simulink model "cap_eq_circuit_pascal5_single_shot"  (R2019a)
settings: Solver=FixedStepAuto  StartTime=0.0  StopTime=sim_time  FixedStep=resolution  MinStep=0.001  RelTol=1e-4  EnableMultiTasking=on
values from neighbouring files (symbols this model uses):
  amps_in = double(amps_in)    [ClassHybrid.m]    (also in Sc.m = double(amps_in_); workspace_test_model.mat = 0)
  capacitance = double(obj.farads)    [ClassHybrid.m]    (also in Sc.m; workspace_test_model.mat = 5)
  resolution = double(resolution)    [ClassHybrid.m]    (also in Sc.m = double(resolution_); matlab.mat = 1; model_out_all.mat = 0.5; workspace_test_model.mat = 10)
  tStep = resolution    (= 0.1)    [ClassHybrid.m]    (also in Sc.m; matlab.mat = 10; model_out_all.mat = 1; raw.mat = 1)
  v_init = ones(x(1), 1, nSeries)    [ClassHybrid.m]    (also in Sc.m; workspace_test_model.mat = [4 4 4 4 4 4 4 4 4 4 4 4 ... (15 elements, 1x5x3)])
libraries: powerlib x127, simulink x5
(part 1 of 2)
settings Model: Creator=ttsh  LastModifiedBy=ttsh
settings SolverCC: ZeroCrossAlgorithm=Adaptive  SolverResetMethod=Robust
settings DataIOCC: LimitDataPoints=on  SaveFormat=Array  ReturnWorkspaceOutputs=off
settings OptimizationCC: LifeSpan=inf
settings DebuggingCC: SolverPrmCheckMsg=warning  UniqueDataStoreMsg=error  AllowSymbolicDim=off  SFUnexpectedBacktrackingDiag=warning  SFNoUnconditionalDefaultTransitionDiag=warning  SFExecutionAtInitializationDiag=none  ArithmeticOperatorsInVariantConditions=warning
settings HardwareCC: ProdBitPerPointer=32  ProdBitPerSizeT=32  ProdBitPerPtrDiffT=32  ProdLargestAtomicFloat=None  ProdIntDivRoundTo=Undefined  ProdEndianess=Unspecified  ProdWordSize=32  ProdHWDeviceType=32-bit Generic
settings ModelReferenceCC: PropagateSignalLabelsOutOfModel=off
settings SFSimCC: SimUseLocalCustomCode=off
settings RTWCC: RTWUseLocalCustomCode=off
settings CodeAppCC: StateflowObjectComments=on
settings GRTTargetCC: TargetLangStandard=C89/C90 (ANSI)  GeneratePreprocessorConditionals=Disable all
settings ConfigComp: CovMetricSettings=dw  CovHtmlReporting=on  CovSaveCumulativeToWorkspaceVar=on  CovSaveSingleToWorkspaceVar=on  CovExternalEMLEnable=off  CovSFcnEnable=off
settings SimscapeCC: SimscapeNormalizeSystem=off

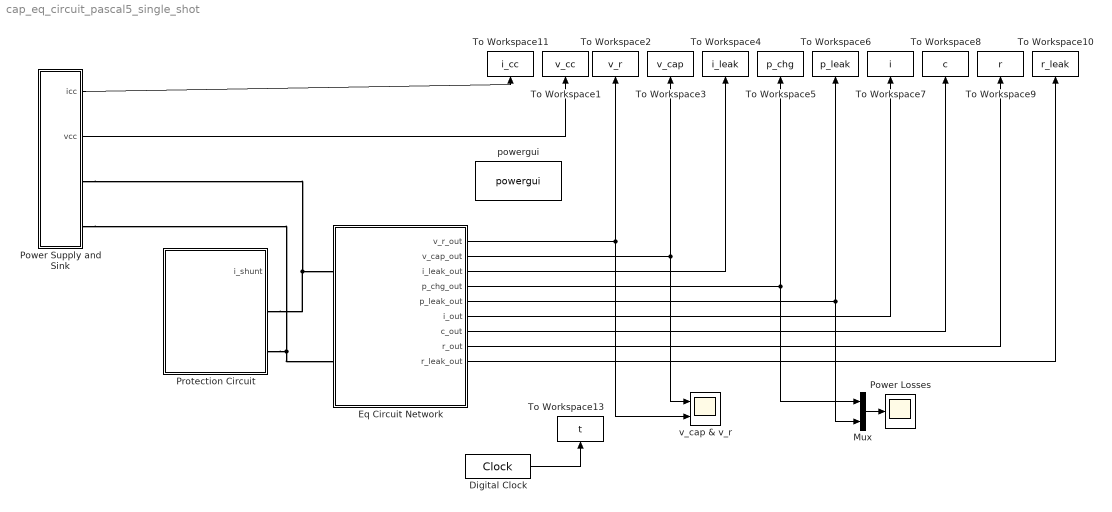
== system cap_eq_circuit_pascal5_single_shot ==
  Digital Clock : DigitalClock  SampleTime=resolution
  Eq Circuit Network : Subsystem  mask{r_leak=inf, c=capacitance, r_esr=0.01, ord=5, v_init1=v_init(1), v_init2=v_init(2), v_init3=v_init(3), v_init4=v_init(4), v_init5=v_init(5)}
      mask prompts: r_leak "R Leak /ohm (inf for disabled)"; c "Capacitance /F"; r_esr "ESR"; ord "Elements (pascal order)"; v_init1 "Initial capacitor voltage"; v_init2 "Initial capacitor voltage"; v_init3 "Initial capacitor voltage"; v_init4 "Initial capacitor voltage"; v_init5 "Initial capacitor voltage"
  Mux : Mux  Inputs=2
  Power Losses : Scope
  Power Supply and Sink : Subsystem  mask{v_ovp=24}
      mask prompts: v_ovp "V OVP"
  Protection Circuit : Subsystem  mask{r=1, d=0.01, v_cut=8.1, v_min=0}
      mask prompts: r "Series resistance"; d "Rate limit"; v_cut "v cutoff"; v_min "v min"
  To Workspace1 : ToWorkspace  VariableName=v_cc  SampleTime=-1
      settings: Save2DSignal=2-D array (concatenate along first dimension)
  To Workspace10 : ToWorkspace  VariableName=r_leak  SampleTime=-1
  To Workspace11 : ToWorkspace  VariableName=i_cc  SampleTime=-1
      settings: Save2DSignal=2-D array (concatenate along first dimension)
  To Workspace13 : ToWorkspace  VariableName=t  SampleTime=-1
      settings: Save2DSignal=2-D array (concatenate along first dimension)
  To Workspace2 : ToWorkspace  VariableName=v_r  SampleTime=-1
  To Workspace3 : ToWorkspace  VariableName=v_cap  SampleTime=-1
  To Workspace4 : ToWorkspace  VariableName=i_leak  SampleTime=-1
  To Workspace5 : ToWorkspace  VariableName=p_chg  SampleTime=-1
  To Workspace6 : ToWorkspace  VariableName=p_leak  SampleTime=-1
  To Workspace7 : ToWorkspace  VariableName=i  SampleTime=-1
  To Workspace8 : ToWorkspace  VariableName=c  SampleTime=-1
  To Workspace9 : ToWorkspace  VariableName=r  SampleTime=-1
  powergui : powerlib/powergui  Priority=1  SimulationMode=Discrete  SampleTime=tStep  frequency=60  Iterations=50  frequencyindice=0  Pbase=100e6  ErrMax=1e-4  UnitsV=V  UnitsW=W  buscounter=0  FunctionMessages=off  echomessages=off  EnableUseOfTLC=off  CurrentSourceSwitches=on  DisableSnubberDevices=on  DisableRonSwitches=off  DisableVfSwitches=off  DisplayEquations=off  AutomaticDiscreteSolvers=off  SolverType=Tustin  Interpol=off  ExternalGateDelay=off  methode=off  Ts=0  x0status=blocks  SPID=on  SwTol=0  HookPort=off  NonlinearTolerance=0  nMaxIteration=15  ContinueOnMaxIteration=off  RestoreLinks=warning  ResistiveCurrentMeasurement=off  Frange=[0:2:500]  Ylog=off  Xlog=on  ShowGrid=off  save=off  variable=ZData  structure=0  ZoomFFT=off  StartTime=0.0  cycles=1  DisplayStyle=1  fundamental=60  FreqAxis=off  MaxFrequency=1000  frequencyindicesteady=1  RmsSteady=1  display=off
      settings: SourceProductName=Simscape Electrical
  v_cap & v_r : Scope  NumInputPorts=2
  wires:
  Eq Circuit Network/1(v_r_out) -> v_cap & v_r/2, To Workspace2/1
  Eq Circuit Network/2(v_cap_out) -> v_cap & v_r/1, To Workspace3/1
  Eq Circuit Network/3(i_leak_out) -> To Workspace4/1
  Eq Circuit Network/4(p_chg_out) -> Mux/1, To Workspace5/1
  Eq Circuit Network/5(p_leak_out) -> Mux/2, To Workspace6/1
  Eq Circuit Network/6(i_out) -> To Workspace7/1
  Eq Circuit Network/7(c_out) -> To Workspace8/1
  Eq Circuit Network/8(r_out) -> To Workspace9/1
  Eq Circuit Network/9(r_leak_out) -> To Workspace10/1
  Mux/1 -> Power Losses/1
  Power Supply and Sink/1(icc) -> To Workspace11/1
  Power Supply and Sink/2(vcc) -> To Workspace1/1
  Digital Clock/1 -> To Workspace13/1
  connections:
  Power Supply and Sink/RConn1 -- Protection Circuit/RConn1 -- Eq Circuit Network/LConn1
  Power Supply and Sink/RConn2 -- Protection Circuit/RConn2 -- Eq Circuit Network/LConn2

== system cap_eq_circuit_pascal5_single_shot/Eq Circuit Network ==
  note: 6x 700R
  note: 4x 1k4
  note: 4x 625R
  note: 1x 550R
  note: 1x 4k
  Subsystem : Subsystem  mask{c=c, r_esr=625, r_leak=r_leak, v_init=v_init2}
      mask prompts: c "Capacitance /F"; r_esr "Series resistance /ohm"; r_leak "Leak resistance /ohm (inf for disabled)"; v_init "Initial capacitor voltage"
  Subsystem1 : Subsystem  mask{c=c, r_esr=1.4e3, r_leak=r_leak, v_init=v_init4}
      mask prompts: c "Capacitance /F"; r_esr "Series resistance /ohm"; r_leak "Leak resistance /ohm (inf for disabled)"; v_init "Initial capacitor voltage"
  Subsystem2 : Subsystem  mask{c=c, r_esr=700, r_leak=r_leak, v_init=v_init3}
      mask prompts: c "Capacitance /F"; r_esr "Series resistance /ohm"; r_leak "Leak resistance /ohm (inf for disabled)"; v_init "Initial capacitor voltage"
  Subsystem5 : Subsystem  mask{c=c, r_esr=4e3, r_leak=r_leak, v_init=v_init5}
      mask prompts: c "Capacitance /F"; r_esr "Series resistance /ohm"; r_leak "Leakage resistance /ohm (inf for disabled)"; v_init "Initial capacitor voltage"
  Subsystem8 : Subsystem  mask{c=c, r_esr=550, r_leak=r_leak, v_init=v_init1}
      mask prompts: c "Capacitance /F"; r_esr "Series resistance /ohm"; r_leak "Leakage resistance /ohm (inf for disabled)"; v_init "Initial capacitor voltage"
  VCC_in : PMIOPort  Side=Left
  VSS_in : PMIOPort  Port=2  Side=Left
  VCC_out : PMIOPort  Port=3  Side=Right
  VSS_out : PMIOPort  Port=4  Side=Right
  v_r_out : Outport
  v_cap_out : Outport  Port=2
  i_leak_out : Outport  Port=3
  p_chg_out : Outport  Port=4
  p_leak_out : Outport  Port=5
  i_out : Outport  Port=6
  c_out : Outport  Port=7
  r_out : Outport  Port=8
  r_leak_out : Outport  Port=9
  wires:
  Subsystem5/5(p_leak_out) -> p_leak_out/1
  Subsystem5/6(i_out) -> i_out/1
  Subsystem5/4(p_chg_out) -> p_chg_out/1
  Subsystem5/7(c_out) -> c_out/1
  Subsystem5/3(i_leak_out) -> i_leak_out/1
  Subsystem5/8(r_out) -> r_out/1
  Subsystem5/2(v_cap_out) -> v_cap_out/1
  Subsystem5/9(r_leak_out) -> r_leak_out/1
  Subsystem5/1(v_r_out) -> v_r_out/1
  Subsystem8/3(i_leak_out) -> Subsystem/3(In3)
  Subsystem8/6(i_out) -> Subsystem/6(In6)
  Subsystem8/9(r_leak_out) -> Subsystem/9(In9)
  Subsystem8/4(p_chg_out) -> Subsystem/4(In4)
  Subsystem8/10(l_out) -> Subsystem/10(In10)
  Subsystem8/8(r_out) -> Subsystem/8(In8)
  Subsystem8/5(p_leak_out) -> Subsystem/5(In5)
  Subsystem8/7(c_out) -> Subsystem/7(In7)
  Subsystem8/1(v_r_out) -> Subsystem/1(In1)
  Subsystem8/2(v_cap_out) -> Subsystem/2(In2)
  Subsystem1/6(Out6) -> Subsystem5/6(i_in)
  Subsystem1/8(Out8) -> Subsystem5/8(r_in)
  Subsystem1/4(Out4) -> Subsystem5/4(p_chg_in)
  Subsystem1/7(Out7) -> Subsystem5/7(c_in)
  Subsystem1/9(Out9) -> Subsystem5/9(r_leak_in)
  Subsystem1/3(Out3) -> Subsystem5/3(i_leak_in)
  Subsystem1/10(Out10) -> Subsystem5/10(l_in)
  Subsystem1/5(Out5) -> Subsystem5/5(p_leak_in)
  Subsystem1/2(Out2) -> Subsystem5/2(v_cap_in)
  Subsystem1/1(Out1) -> Subsystem5/1(v_r_in)
  Subsystem/3(Out3) -> Subsystem2/3(In3)
  Subsystem/10(Out10) -> Subsystem2/10(In10)
  Subsystem/8(Out8) -> Subsystem2/8(In8)
  Subsystem/1(Out1) -> Subsystem2/1(In1)
  Subsystem/2(Out2) -> Subsystem2/2(In2)
  Subsystem/6(Out6) -> Subsystem2/6(In6)
  Subsystem/9(Out9) -> Subsystem2/9(In9)
  Subsystem/7(Out7) -> Subsystem2/7(In7)
  Subsystem/4(Out4) -> Subsystem2/4(In4)
  Subsystem/5(Out5) -> Subsystem2/5(In5)
  Subsystem2/5(Out5) -> Subsystem1/5(In5)
  Subsystem2/8(Out8) -> Subsystem1/8(In8)
  Subsystem2/6(Out6) -> Subsystem1/6(In6)
  Subsystem2/2(Out2) -> Subsystem1/2(In2)
  Subsystem2/10(Out10) -> Subsystem1/10(In10)
  Subsystem2/9(Out9) -> Subsystem1/9(In9)
  Subsystem2/1(Out1) -> Subsystem1/1(In1)
  Subsystem2/3(Out3) -> Subsystem1/3(In3)
  Subsystem2/4(Out4) -> Subsystem1/4(In4)
  Subsystem2/7(Out7) -> Subsystem1/7(In7)
  connections:
  Subsystem8/LConn1 -- VCC_in/RConn1
  VSS_in/RConn1 -- Subsystem8/LConn2
  Subsystem8/RConn2 -- Subsystem/LConn2
  Subsystem8/RConn1 -- Subsystem/LConn1
  Subsystem1/RConn2 -- Subsystem5/LConn2
  Subsystem1/RConn1 -- Subsystem5/LConn1
  Subsystem/RConn1 -- Subsystem2/LConn1
  Subsystem/RConn2 -- Subsystem2/LConn2
  Subsystem1/LConn2 -- Subsystem2/RConn2
  Subsystem1/LConn1 -- Subsystem2/RConn1
  VCC_out/RConn1 -- Subsystem5/RConn1
  Subsystem5/RConn2 -- VSS_out/RConn1

== system cap_eq_circuit_pascal5_single_shot/Power Supply and Sink ==
  Compare To Zero : simulink/Logic and Bit Operations/Compare To Zero  relop=>  OutDataTypeStr=boolean
  Compare To Zero1 : simulink/Logic and Bit Operations/Compare To Zero  relop=~=  OutDataTypeStr=boolean
  Constant : Constant  Value=3*5
  Constant1 : Constant  Value=amps_in
  Controlled Current Source2 : powerlib/Electrical Sources/Controlled Current Source  Initialize=on  Source_Type=DC  Amplitude=0  Phase=0  Frequency=0  Measurements=None
      settings: SourceProductName=Simscape Electrical
  Discrete PID Controller : simulink/Continuous/PID Controller  Controller=PI  Form=Parallel  TimeDomain=Discrete-time  SampleTime=-1  IntegratorMethod=Forward Euler  FilterMethod=Forward Euler  ControllerParametersSource=internal  P=1  I=0.02  D=0  UseFilter=on  N=100  TunerSelectOption=Transfer Function Based (PID Tuner App)  InitialConditionSource=internal  InitialConditionForIntegrator=0  InitialConditionForFilter=0  DifferentiatorICPrevScaledInput=0  ExternalReset=none  TrackingMode=off  Kt=1  LimitOutput=on  UpperSaturationLimit=0.1  LowerSaturationLimit=0  LinearizeAsGain=off  AntiWindupMode=none  Kb=1  POutMin=[]  POutMax=[]  IOutMin=[]  IOutMax=[]  DOutMin=[]  DOutMax=[]  NOutMin=[]  NOutMax=[]  SumOutMin=[]  SumOutMax=[]  SaturationOutMin=[]  SaturationOutMax=[]  PParamMin=[]  PParamMax=[]  IParamMin=[]  IParamMax=[]  DParamMin=[]  DParamMax=[]  NParamMin=[]  NParamMax=[]  KbParamMin=[]  KbParamMax=[]  KtParamMin=[]  KtParamMax=[]  KbOutMin=[]  KbOutMax=[]  KtOutMin=[]  KtOutMax=[]  IntegratorOutMin=[]  IntegratorOutMax=[]  FilterOutMin=[]  FilterOutMax=[]  SumI1OutMin=[]  SumI1OutMax=[]  SumI2OutMin=[]  SumI2OutMax=[]  SumI3OutMin=[]  SumI3OutMax=[]  SumI4OutMin=[]  SumI4OutMax=[]  SumDOutMin=[]  SumDOutMax=[]  DifferentiatorOutMin=[]  DifferentiatorOutMax=[]  FilterDiffOutCoefMin=[]  FilterDiffOutCoefMax=[]  ReciprocalOutMin=[]  ReciprocalOutMax=[]  SumDenOutMin=[]  SumDenOutMax=[]  SumNumOutMin=[]  SumNumOutMax=[]  DivideOutMin=[]  DivideOutMax=[]  IntegratorContinuousStateAttributes=''  IntegratorStateMustResolveToSignalObject=off  IntegratorRTWStateStorageClass=Auto  FilterContinuousStateAttributes=''  FilterStateMustResolveToSignalObject=off  FilterRTWStateStorageClass=Auto  ParallelPVariant=InternalParameters  IdealPVariant=Disabled  IVariant=InternalParameters  DVariant=Disabled  IntegratorVariant=Discrete  SatVariant=Enabled  AWVariant=Passthrough  PCopyVariant=Disabled  TRVariant=Disabled  FdbkBlocksVariant=Forward  IdealPFdbkVariant=Disabled  SatFdbkVariant=Disabled  DerivativeFilterVariant=Disabled  NVariant=Disabled  NCopyVariant=Disabled_SignalSpec  FilterICVariant=Disabled  IntegratorICVariant=InternalICs  ExternalResetVariant=Disabled  TRSumVariant=Passthrough  SumFdbkVariant=Disabled  SumVariant=Sum_PI
  Display : Display
  Memory : Memory  InitialCondition=1  InheritSampleTime=on  LinearizeAsDelay=on
  Mosfet : powerlib/Power Electronics/Mosfet  Ron=0.1  Lon=0  Rd=0.01  Vfd=0  IC=0  Rs=1e5  Cs=inf  Measurements=off
      settings: SourceProductName=Simscape Electrical
  Mosfet1 : powerlib/Power Electronics/Mosfet  Ron=0.1  Lon=0  Rd=0.01  Vfd=0  IC=0  Rs=1e5  Cs=inf  Measurements=off
      settings: SourceProductName=Simscape Electrical
  Saturation : Saturate  UpperLimit=inf  LowerLimit=0
  Series RLC Branch : powerlib/Elements/Series RLC Branch  LConnTagsString=__new0  RConnTagsString=__new0  BranchType=R  Resistance=0.001  Inductance=1e-9  SetiL0=off  InitialCurrent=0  Capacitance=1e-6  Setx0=off  InitialVoltage=0  Measurements=None
      settings: SourceProductName=Simscape Electrical
  Series RLC Branch1 : powerlib/Elements/Series RLC Branch  LConnTagsString=__new0  RConnTagsString=__new0  BranchType=R  Resistance=1e9  Inductance=1e-9  SetiL0=off  InitialCurrent=0  Capacitance=1e-6  Setx0=off  InitialVoltage=0  Measurements=None
      settings: SourceProductName=Simscape Electrical
  Series RLC Branch2 : powerlib/Elements/Series RLC Branch  LConnTagsString=__new0  RConnTagsString=__new0  BranchType=R  Resistance=1e9  Inductance=1e-9  SetiL0=off  InitialCurrent=0  Capacitance=1e-6  Setx0=off  InitialVoltage=0  Measurements=None
      settings: SourceProductName=Simscape Electrical
  Sum : Sum  Inputs=|-+
  Switch : Switch  Criteria=u2 > Threshold
  i_cc : powerlib/Measurements/Current Measurement  PhasorSimulation=off  OutputType=Complex  PSBequivalent=0
      settings: SourceProductName=Simscape Electrical
  v_cap_single1 : powerlib/Measurements/Voltage Measurement  PhasorSimulation=off  OutputType=Complex  PSBequivalent=0
      settings: SourceProductName=Simscape Electrical
  V_cc : PMIOPort  Side=Right
  V_ss : PMIOPort  Port=2  Side=Right
  icc : Outport
  vcc : Outport  Port=2
  wires:
  Saturation/1 -> Switch/3
  Compare To Zero1/1 -> Mosfet1/1, Mosfet/1
  i_cc/1 -> icc/1
  v_cap_single1/1 -> vcc/1, [vcc]
  [vcc] -> Sum/1, Compare To Zero/1
  Memory/1 -> Switch/2
  Compare To Zero/1 -> Memory/1
  Switch/1 -> Controlled Current Source2/1
  Sum/1 -> Discrete PID Controller/1
  Constant1/1 -> Saturation/1, Compare To Zero1/1, Switch/1
  Constant/1 -> Sum/2
  Discrete PID Controller/1 -> Display/1
  connections:
  Mosfet/LConn1 -- Mosfet1/LConn1
  Mosfet1/RConn1 -- Series RLC Branch2/LConn1 -- Controlled Current Source2/RConn1
  i_cc/LConn1 -- V_cc/RConn1
  i_cc/RConn1 -- Mosfet/RConn1 -- Series RLC Branch1/LConn1 -- v_cap_single1/LConn1
  Controlled Current Source2/LConn1 -- Series RLC Branch/LConn1
  v_cap_single1/LConn2 -- Series RLC Branch2/RConn1 -- Series RLC Branch/RConn1 -- Series RLC Branch1/RConn1 -- V_ss/RConn1

== system cap_eq_circuit_pascal5_single_shot/Protection Circuit ==
  note: 10nF
  Compare To Constant : simulink/Logic and Bit Operations/Compare To Constant  relop=>  const=v_cut  OutDataTypeStr=boolean
  Compare To Constant1 : simulink/Logic and Bit Operations/Compare To Constant  relop=<  const=v_min  OutDataTypeStr=boolean
  Mosfet : powerlib/Power Electronics/Mosfet  Ron=0.1  Lon=0  Rd=0.01  Vfd=0  IC=0  Rs=1e5  Cs=inf  Measurements=off
      settings: SourceProductName=Simscape Electrical
  Mosfet1 : powerlib/Power Electronics/Mosfet  Ron=0.1  Lon=0  Rd=0.01  Vfd=0  IC=0  Rs=1e5  Cs=inf  Measurements=off
      settings: SourceProductName=Simscape Electrical
  Parallel RLC Branch11 : powerlib/Elements/Parallel RLC Branch  LConnTagsString=a  RConnTagsString=__new0  BranchType=C  Resistance=1  Inductance=1e-3  SetiL0=off  InitialCurrent=0  Capacitance=0.00000001  Setx0=on  InitialVoltage=1.0  Measurements=None
      settings: SourceProductName=Simscape Electrical
  Series RLC Branch1 : powerlib/Elements/Series RLC Branch  LConnTagsString=__new0  RConnTagsString=__new0  BranchType=R  Resistance=r  Inductance=1e-3  SetiL0=off  InitialCurrent=0  Capacitance=1e-6  Setx0=off  InitialVoltage=0  Measurements=None
      settings: SourceProductName=Simscape Electrical
  Sum : Sum  Inputs=++|
  i_cc : powerlib/Measurements/Current Measurement  PhasorSimulation=off  OutputType=Complex  PSBequivalent=0
      settings: SourceProductName=Simscape Electrical
  v_cap_single2 : powerlib/Measurements/Voltage Measurement  PhasorSimulation=off  OutputType=Complex  PSBequivalent=0
      settings: SourceProductName=Simscape Electrical
  vcc : PMIOPort  Side=Right
  vss : PMIOPort  Port=2  Side=Right
  i_shunt : Outport
  wires:
  i_cc/1 -> i_shunt/1
  v_cap_single2/1 -> Compare To Constant1/1, Compare To Constant/1
  Compare To Constant/1 -> Sum/2
  Compare To Constant1/1 -> Sum/1
  Sum/1 -> Mosfet/1, Mosfet1/1
  connections:
  Series RLC Branch1/LConn1 -- i_cc/LConn1
  i_cc/RConn1 -- Mosfet/RConn1
  Mosfet1/LConn1 -- Mosfet/LConn1
  vcc/RConn1 -- Mosfet1/RConn1 -- Parallel RLC Branch11/LConn1 -- v_cap_single2/LConn1
  v_cap_single2/LConn2 -- Parallel RLC Branch11/RConn1 -- vss/RConn1 -- Series RLC Branch1/RConn1

== system cap_eq_circuit_pascal5_single_shot/Eq Circuit Network/Subsystem ==
  In1 : Inport
  In2 : Inport  Port=2
  In3 : Inport  Port=3
  In4 : Inport  Port=4
  In5 : Inport  Port=5
  In6 : Inport  Port=6
  In7 : Inport  Port=7
  In8 : Inport  Port=8
  In9 : Inport  Port=9
  In10 : Inport  Port=10
  Subsystem1 : Subsystem  mask{c=c, r_esr=r_esr, r_leak=r_leak, v_init=v_init}
      mask prompts: c "Capacitance /F"; r_esr "Series resistance /ohm"; r_leak "Leakage resistance /ohm (inf for disabled)"; v_init "Initial capacitor voltage"
  Subsystem2 : Subsystem  mask{c=c, r_esr=r_esr, r_leak=r_leak, v_init=v_init}
      mask prompts: c "Capacitance /F"; r_esr "Series resistance /ohm"; r_leak "Leakage resistance /ohm (inf for disabled)"; v_init "Initial capacitor voltage"
  Subsystem3 : Subsystem  mask{c=c, r_esr=r_esr, r_leak=r_leak, v_init=v_init}
      mask prompts: c "Capacitance /F"; r_esr "Series resistance /ohm"; r_leak "Leakage resistance /ohm (inf for disabled)"; v_init "Initial capacitor voltage"
  Subsystem5 : Subsystem  mask{c=c, r_esr=r_esr, r_leak=r_leak, v_init=v_init}
      mask prompts: c "Capacitance /F"; r_esr "Series resistance /ohm"; r_leak "Leakage resistance /ohm (inf for disabled)"; v_init "Initial capacitor voltage"
  Conn1 : PMIOPort  Side=Left
  Conn2 : PMIOPort  Port=2  Side=Right
  Conn3 : PMIOPort  Port=3  Side=Left
  Conn4 : PMIOPort  Port=4  Side=Right
  Out1 : Outport
  Out2 : Outport  Port=2
  Out3 : Outport  Port=3
  Out4 : Outport  Port=4
  Out5 : Outport  Port=5
  Out6 : Outport  Port=6
  Out7 : Outport  Port=7
  Out8 : Outport  Port=8
  Out9 : Outport  Port=9
  Out10 : Outport  Port=10
  wires:
  In8/1 -> Subsystem5/8(r_in)
  In3/1 -> Subsystem5/3(i_leak_in)
  In10/1 -> Subsystem5/10(l_in)
  In1/1 -> Subsystem5/1(v_r_in)
  In7/1 -> Subsystem5/7(c_in)
  In4/1 -> Subsystem5/4(p_chg_in)
  In5/1 -> Subsystem5/5(p_leak_in)
  In6/1 -> Subsystem5/6(i_in)
  In9/1 -> Subsystem5/9(r_leak_in)
  In2/1 -> Subsystem5/2(v_cap_in)
  Subsystem5/1(v_r_out) -> Subsystem1/1(v_r_in)
  Subsystem5/2(v_cap_out) -> Subsystem1/2(v_cap_in)
  Subsystem5/3(i_leak_out) -> Subsystem1/3(i_leak_in)
  Subsystem5/4(p_chg_out) -> Subsystem1/4(p_chg_in)
  Subsystem5/5(p_leak_out) -> Subsystem1/5(p_leak_in)
  Subsystem5/6(i_out) -> Subsystem1/6(i_in)
  Subsystem5/7(c_out) -> Subsystem1/7(c_in)
  Subsystem5/8(r_out) -> Subsystem1/8(r_in)
  Subsystem5/9(r_leak_out) -> Subsystem1/9(r_leak_in)
  Subsystem5/10(l_out) -> Subsystem1/10(l_in)
  Subsystem1/1(v_r_out) -> Subsystem2/1(v_r_in)
  Subsystem1/2(v_cap_out) -> Subsystem2/2(v_cap_in)
  Subsystem1/3(i_leak_out) -> Subsystem2/3(i_leak_in)
  Subsystem1/4(p_chg_out) -> Subsystem2/4(p_chg_in)
  Subsystem1/5(p_leak_out) -> Subsystem2/5(p_leak_in)
  Subsystem1/6(i_out) -> Subsystem2/6(i_in)
  Subsystem1/7(c_out) -> Subsystem2/7(c_in)
  Subsystem1/8(r_out) -> Subsystem2/8(r_in)
  Subsystem1/9(r_leak_out) -> Subsystem2/9(r_leak_in)
  Subsystem1/10(l_out) -> Subsystem2/10(l_in)
  Subsystem2/1(v_r_out) -> Subsystem3/1(v_r_in)
  Subsystem3/1(v_r_out) -> Out1/1
  Subsystem2/2(v_cap_out) -> Subsystem3/2(v_cap_in)
  Subsystem2/3(i_leak_out) -> Subsystem3/3(i_leak_in)
  Subsystem2/4(p_chg_out) -> Subsystem3/4(p_chg_in)
  Subsystem2/5(p_leak_out) -> Subsystem3/5(p_leak_in)
  Subsystem2/6(i_out) -> Subsystem3/6(i_in)
  Subsystem2/7(c_out) -> Subsystem3/7(c_in)
  Subsystem2/8(r_out) -> Subsystem3/8(r_in)
  Subsystem2/9(r_leak_out) -> Subsystem3/9(r_leak_in)
  Subsystem2/10(l_out) -> Subsystem3/10(l_in)
  Subsystem3/2(v_cap_out) -> Out2/1
  Subsystem3/3(i_leak_out) -> Out3/1
  Subsystem3/4(p_chg_out) -> Out4/1
  Subsystem3/5(p_leak_out) -> Out5/1
  Subsystem3/6(i_out) -> Out6/1
  Subsystem3/7(c_out) -> Out7/1
  Subsystem3/8(r_out) -> Out8/1
  Subsystem3/9(r_leak_out) -> Out9/1
  Subsystem3/10(l_out) -> Out10/1
  connections:
  Subsystem5/LConn2 -- Conn3/RConn1
  Subsystem5/LConn1 -- Conn1/RConn1
  Subsystem1/LConn1 -- Subsystem5/RConn1
  Subsystem1/LConn2 -- Subsystem5/RConn2
  Subsystem2/LConn1 -- Subsystem1/RConn1
  Subsystem2/LConn2 -- Subsystem1/RConn2
  Subsystem3/LConn1 -- Subsystem2/RConn1
  Subsystem3/LConn2 -- Subsystem2/RConn2
  Subsystem3/RConn1 -- Conn2/RConn1
  Subsystem3/RConn2 -- Conn4/RConn1

== system cap_eq_circuit_pascal5_single_shot/Eq Circuit Network/Subsystem1 ==
  In1 : Inport
  In2 : Inport  Port=2
  In3 : Inport  Port=3
  In4 : Inport  Port=4
  In5 : Inport  Port=5
  In6 : Inport  Port=6
  In7 : Inport  Port=7
  In8 : Inport  Port=8
  In9 : Inport  Port=9
  In10 : Inport  Port=10
  Subsystem1 : Subsystem  mask{c=c, r_esr=r_esr, r_leak=r_leak, v_init=v_init}
      mask prompts: c "Capacitance /F"; r_esr "Series resistance /ohm"; r_leak "Leakage resistance /ohm (inf for disabled)"; v_init "Initial capacitor voltage"
  Subsystem2 : Subsystem  mask{c=c, r_esr=r_esr, r_leak=r_leak, v_init=v_init}
      mask prompts: c "Capacitance /F"; r_esr "Series resistance /ohm"; r_leak "Leakage resistance /ohm (inf for disabled)"; v_init "Initial capacitor voltage"
  Subsystem3 : Subsystem  mask{c=c, r_esr=r_esr, r_leak=r_leak, v_init=v_init}
      mask prompts: c "Capacitance /F"; r_esr "Series resistance /ohm"; r_leak "Leakage resistance /ohm (inf for disabled)"; v_init "Initial capacitor voltage"
  Subsystem5 : Subsystem  mask{c=c, r_esr=r_esr, r_leak=r_leak, v_init=v_init}
      mask prompts: c "Capacitance /F"; r_esr "Series resistance /ohm"; r_leak "Leakage resistance /ohm (inf for disabled)"; v_init "Initial capacitor voltage"
  Conn1 : PMIOPort  Side=Left
  Conn2 : PMIOPort  Port=2  Side=Right
  Conn3 : PMIOPort  Port=3  Side=Left
  Conn4 : PMIOPort  Port=4  Side=Right
  Out1 : Outport
  Out2 : Outport  Port=2
  Out3 : Outport  Port=3
  Out4 : Outport  Port=4
  Out5 : Outport  Port=5
  Out6 : Outport  Port=6
  Out7 : Outport  Port=7
  Out8 : Outport  Port=8
  Out9 : Outport  Port=9
  Out10 : Outport  Port=10
  wires:
  Subsystem3/10(l_out) -> Out10/1
  Subsystem3/9(r_leak_out) -> Out9/1
  Subsystem3/8(r_out) -> Out8/1
  Subsystem3/7(c_out) -> Out7/1
  Subsystem3/6(i_out) -> Out6/1
  Subsystem3/5(p_leak_out) -> Out5/1
  Subsystem3/4(p_chg_out) -> Out4/1
  Subsystem3/3(i_leak_out) -> Out3/1
  Subsystem3/2(v_cap_out) -> Out2/1
  Subsystem2/10(l_out) -> Subsystem3/10(l_in)
  Subsystem2/9(r_leak_out) -> Subsystem3/9(r_leak_in)
  Subsystem2/8(r_out) -> Subsystem3/8(r_in)
  Subsystem2/7(c_out) -> Subsystem3/7(c_in)
  Subsystem2/6(i_out) -> Subsystem3/6(i_in)
  Subsystem2/5(p_leak_out) -> Subsystem3/5(p_leak_in)
  Subsystem2/4(p_chg_out) -> Subsystem3/4(p_chg_in)
  Subsystem2/3(i_leak_out) -> Subsystem3/3(i_leak_in)
  Subsystem2/2(v_cap_out) -> Subsystem3/2(v_cap_in)
  Subsystem3/1(v_r_out) -> Out1/1
  Subsystem2/1(v_r_out) -> Subsystem3/1(v_r_in)
  Subsystem1/10(l_out) -> Subsystem2/10(l_in)
  Subsystem1/9(r_leak_out) -> Subsystem2/9(r_leak_in)
  Subsystem1/8(r_out) -> Subsystem2/8(r_in)
  Subsystem1/7(c_out) -> Subsystem2/7(c_in)
  Subsystem1/6(i_out) -> Subsystem2/6(i_in)
  Subsystem1/5(p_leak_out) -> Subsystem2/5(p_leak_in)
  Subsystem1/4(p_chg_out) -> Subsystem2/4(p_chg_in)
  Subsystem1/3(i_leak_out) -> Subsystem2/3(i_leak_in)
  Subsystem1/2(v_cap_out) -> Subsystem2/2(v_cap_in)
  Subsystem1/1(v_r_out) -> Subsystem2/1(v_r_in)
  Subsystem5/10(l_out) -> Subsystem1/10(l_in)
  Subsystem5/9(r_leak_out) -> Subsystem1/9(r_leak_in)
  Subsystem5/8(r_out) -> Subsystem1/8(r_in)
  Subsystem5/7(c_out) -> Subsystem1/7(c_in)
  Subsystem5/6(i_out) -> Subsystem1/6(i_in)
  Subsystem5/5(p_leak_out) -> Subsystem1/5(p_leak_in)
  Subsystem5/4(p_chg_out) -> Subsystem1/4(p_chg_in)
  Subsystem5/3(i_leak_out) -> Subsystem1/3(i_leak_in)
  Subsystem5/2(v_cap_out) -> Subsystem1/2(v_cap_in)
  Subsystem5/1(v_r_out) -> Subsystem1/1(v_r_in)
  In2/1 -> Subsystem5/2(v_cap_in)
  In9/1 -> Subsystem5/9(r_leak_in)
  In6/1 -> Subsystem5/6(i_in)
  In5/1 -> Subsystem5/5(p_leak_in)
  In4/1 -> Subsystem5/4(p_chg_in)
  In7/1 -> Subsystem5/7(c_in)
  In1/1 -> Subsystem5/1(v_r_in)
  In10/1 -> Subsystem5/10(l_in)
  In3/1 -> Subsystem5/3(i_leak_in)
  In8/1 -> Subsystem5/8(r_in)
  connections:
  Subsystem3/RConn2 -- Conn4/RConn1
  Subsystem3/RConn1 -- Conn2/RConn1
  Subsystem3/LConn2 -- Subsystem2/RConn2
  Subsystem3/LConn1 -- Subsystem2/RConn1
  Subsystem2/LConn2 -- Subsystem1/RConn2
  Subsystem2/LConn1 -- Subsystem1/RConn1
  Subsystem1/LConn2 -- Subsystem5/RConn2
  Subsystem1/LConn1 -- Subsystem5/RConn1
  Subsystem5/LConn1 -- Conn1/RConn1
  Subsystem5/LConn2 -- Conn3/RConn1

== system cap_eq_circuit_pascal5_single_shot/Eq Circuit Network/Subsystem2 ==
  In1 : Inport
  In2 : Inport  Port=2
  In3 : Inport  Port=3
  In4 : Inport  Port=4
  In5 : Inport  Port=5
  In6 : Inport  Port=6
  In7 : Inport  Port=7
  In8 : Inport  Port=8
  In9 : Inport  Port=9
  In10 : Inport  Port=10
  Subsystem1 : Subsystem  mask{c=c, r_esr=r_esr, r_leak=r_leak, v_init=v_init}
      mask prompts: c "Capacitance /F"; r_esr "Series resistance /ohm"; r_leak "Leakage resistance /ohm (inf for disabled)"; v_init "Initial capacitor voltage"
  Subsystem2 : Subsystem  mask{c=c, r_esr=r_esr, r_leak=r_leak, v_init=v_init}
      mask prompts: c "Capacitance /F"; r_esr "Series resistance /ohm"; r_leak "Leakage resistance /ohm (inf for disabled)"; v_init "Initial capacitor voltage"
  Subsystem3 : Subsystem  mask{c=c, r_esr=r_esr, r_leak=r_leak, v_init=v_init}
      mask prompts: c "Capacitance /F"; r_esr "Series resistance /ohm"; r_leak "Leakage resistance /ohm (inf for disabled)"; v_init "Initial capacitor voltage"
  Subsystem4 : Subsystem  mask{c=c, r_esr=r_esr, r_leak=r_leak, v_init=v_init}
      mask prompts: c "Capacitance /F"; r_esr "Series resistance /ohm"; r_leak "Leakage resistance /ohm (inf for disabled)"; v_init "Initial capacitor voltage"
  Subsystem5 : Subsystem  mask{c=c, r_esr=r_esr, r_leak=r_leak, v_init=v_init}
      mask prompts: c "Capacitance /F"; r_esr "Series resistance /ohm"; r_leak "Leakage resistance /ohm (inf for disabled)"; v_init "Initial capacitor voltage"
  Subsystem6 : Subsystem  mask{c=c, r_esr=r_esr, r_leak=r_leak, v_init=v_init}
      mask prompts: c "Capacitance /F"; r_esr "Series resistance /ohm"; r_leak "Leakage resistance /ohm (inf for disabled)"; v_init "Initial capacitor voltage"
  Conn1 : PMIOPort  Side=Left
  Conn2 : PMIOPort  Port=2  Side=Right
  Conn3 : PMIOPort  Port=3  Side=Left
  Conn4 : PMIOPort  Port=4  Side=Right
  Out1 : Outport
  Out2 : Outport  Port=2
  Out3 : Outport  Port=3
  Out4 : Outport  Port=4
  Out5 : Outport  Port=5
  Out6 : Outport  Port=6
  Out7 : Outport  Port=7
  Out8 : Outport  Port=8
  Out9 : Outport  Port=9
  Out10 : Outport  Port=10
  wires:
  In1/1 -> Subsystem5/1(v_r_in)
  In2/1 -> Subsystem5/2(v_cap_in)
  In3/1 -> Subsystem5/3(i_leak_in)
  In4/1 -> Subsystem5/4(p_chg_in)
  In5/1 -> Subsystem5/5(p_leak_in)
  In6/1 -> Subsystem5/6(i_in)
  In7/1 -> Subsystem5/7(c_in)
  In8/1 -> Subsystem5/8(r_in)
  In9/1 -> Subsystem5/9(r_leak_in)
  In10/1 -> Subsystem5/10(l_in)
  Subsystem5/1(v_r_out) -> Subsystem1/1(v_r_in)
  Subsystem5/2(v_cap_out) -> Subsystem1/2(v_cap_in)
  Subsystem5/3(i_leak_out) -> Subsystem1/3(i_leak_in)
  Subsystem5/4(p_chg_out) -> Subsystem1/4(p_chg_in)
  Subsystem5/5(p_leak_out) -> Subsystem1/5(p_leak_in)
  Subsystem5/6(i_out) -> Subsystem1/6(i_in)
  Subsystem5/7(c_out) -> Subsystem1/7(c_in)
  Subsystem5/8(r_out) -> Subsystem1/8(r_in)
  Subsystem5/9(r_leak_out) -> Subsystem1/9(r_leak_in)
  Subsystem5/10(l_out) -> Subsystem1/10(l_in)
  Subsystem1/1(v_r_out) -> Subsystem2/1(v_r_in)
  Subsystem1/2(v_cap_out) -> Subsystem2/2(v_cap_in)
  Subsystem1/3(i_leak_out) -> Subsystem2/3(i_leak_in)
  Subsystem1/4(p_chg_out) -> Subsystem2/4(p_chg_in)
  Subsystem1/5(p_leak_out) -> Subsystem2/5(p_leak_in)
  Subsystem1/6(i_out) -> Subsystem2/6(i_in)
  Subsystem1/7(c_out) -> Subsystem2/7(c_in)
  Subsystem1/8(r_out) -> Subsystem2/8(r_in)
  Subsystem1/9(r_leak_out) -> Subsystem2/9(r_leak_in)
  Subsystem1/10(l_out) -> Subsystem2/10(l_in)
  Subsystem2/1(v_r_out) -> Subsystem3/1(v_r_in)
  Subsystem2/2(v_cap_out) -> Subsystem3/2(v_cap_in)
  Subsystem2/3(i_leak_out) -> Subsystem3/3(i_leak_in)
  Subsystem2/4(p_chg_out) -> Subsystem3/4(p_chg_in)
  Subsystem2/5(p_leak_out) -> Subsystem3/5(p_leak_in)
  Subsystem2/6(i_out) -> Subsystem3/6(i_in)
  Subsystem2/7(c_out) -> Subsystem3/7(c_in)
  Subsystem2/8(r_out) -> Subsystem3/8(r_in)
  Subsystem2/9(r_leak_out) -> Subsystem3/9(r_leak_in)
  Subsystem2/10(l_out) -> Subsystem3/10(l_in)
  Subsystem3/1(v_r_out) -> Subsystem4/1(v_r_in)
  Subsystem3/2(v_cap_out) -> Subsystem4/2(v_cap_in)
  Subsystem3/3(i_leak_out) -> Subsystem4/3(i_leak_in)
  Subsystem3/4(p_chg_out) -> Subsystem4/4(p_chg_in)
  Subsystem3/5(p_leak_out) -> Subsystem4/5(p_leak_in)
  Subsystem3/6(i_out) -> Subsystem4/6(i_in)
  Subsystem3/7(c_out) -> Subsystem4/7(c_in)
  Subsystem3/8(r_out) -> Subsystem4/8(r_in)
  Subsystem3/9(r_leak_out) -> Subsystem4/9(r_leak_in)
  Subsystem3/10(l_out) -> Subsystem4/10(l_in)
  Subsystem4/1(v_r_out) -> Subsystem6/1(v_r_in)
  Subsystem4/2(v_cap_out) -> Subsystem6/2(v_cap_in)
  Subsystem4/3(i_leak_out) -> Subsystem6/3(i_leak_in)
  Subsystem4/4(p_chg_out) -> Subsystem6/4(p_chg_in)
  Subsystem4/5(p_leak_out) -> Subsystem6/5(p_leak_in)
  Subsystem4/6(i_out) -> Subsystem6/6(i_in)
  Subsystem4/7(c_out) -> Subsystem6/7(c_in)
  Subsystem4/8(r_out) -> Subsystem6/8(r_in)
  Subsystem4/9(r_leak_out) -> Subsystem6/9(r_leak_in)
  Subsystem4/10(l_out) -> Subsystem6/10(l_in)
  Subsystem6/1(v_r_out) -> Out1/1
  Subsystem6/2(v_cap_out) -> Out2/1
  Subsystem6/3(i_leak_out) -> Out3/1
  Subsystem6/4(p_chg_out) -> Out4/1
  Subsystem6/5(p_leak_out) -> Out5/1
  Subsystem6/6(i_out) -> Out6/1
  Subsystem6/7(c_out) -> Out7/1
  Subsystem6/8(r_out) -> Out8/1
  Subsystem6/9(r_leak_out) -> Out9/1
  Subsystem6/10(l_out) -> Out10/1
  connections:
  Conn1/RConn1 -- Subsystem5/LConn1
  Conn3/RConn1 -- Subsystem5/LConn2
  Subsystem1/LConn1 -- Subsystem5/RConn1
  Subsystem1/LConn2 -- Subsystem5/RConn2
  Subsystem2/LConn1 -- Subsystem1/RConn1
  Subsystem2/LConn2 -- Subsystem1/RConn2
  Subsystem3/LConn1 -- Subsystem2/RConn1
  Subsystem3/LConn2 -- Subsystem2/RConn2
  Subsystem4/LConn1 -- Subsystem3/RConn1
  Subsystem4/LConn2 -- Subsystem3/RConn2
  Subsystem6/LConn1 -- Subsystem4/RConn1
  Subsystem6/LConn2 -- Subsystem4/RConn2
  Subsystem6/RConn1 -- Conn2/RConn1
  Subsystem6/RConn2 -- Conn4/RConn1

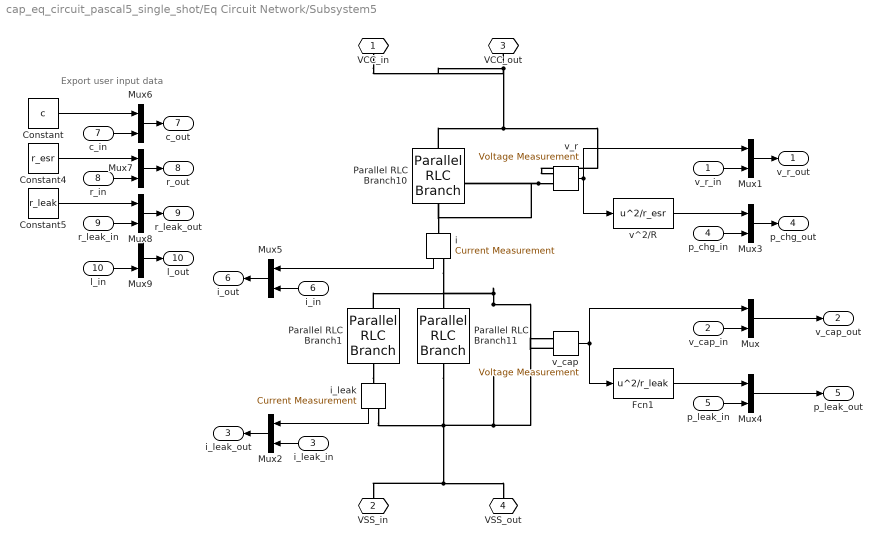
== system cap_eq_circuit_pascal5_single_shot/Eq Circuit Network/Subsystem5 ==
  note: Export user input data
  v_r_in : Inport
  v_cap_in : Inport  Port=2
  i_leak_in : Inport  Port=3
  p_chg_in : Inport  Port=4
  p_leak_in : Inport  Port=5
  i_in : Inport  Port=6
  c_in : Inport  Port=7
  r_in : Inport  Port=8
  r_leak_in : Inport  Port=9
  l_in : Inport  Port=10
  Constant : Constant  Value=c
  Constant4 : Constant  Value=r_esr
  Constant5 : Constant  Value=r_leak
  Fcn1 : Fcn  Expr=u^2/r_leak
  Mux{,1..9} (10 alike) : Mux  Inputs=2
  Parallel RLC Branch1 : powerlib/Elements/Parallel RLC Branch  LConnTagsString=a  RConnTagsString=__new0  BranchType=R  Resistance=r_esr  Inductance=1e-3  SetiL0=off  InitialCurrent=0  Capacitance=1e-6  Setx0=off  InitialVoltage=0  Measurements=None
      settings: SourceProductName=Simscape Electrical
  Parallel RLC Branch10 : powerlib/Elements/Parallel RLC Branch  LConnTagsString=a  RConnTagsString=__new0  BranchType=R  Resistance=r_esr  Inductance=1e-3  SetiL0=off  InitialCurrent=0  Capacitance=1e-6  Setx0=off  InitialVoltage=0  Measurements=None
      settings: SourceProductName=Simscape Electrical
  Parallel RLC Branch11 : powerlib/Elements/Parallel RLC Branch  LConnTagsString=a  RConnTagsString=__new0  BranchType=C  Resistance=1  Inductance=1e-3  SetiL0=off  InitialCurrent=0  Capacitance=c  Setx0=on  InitialVoltage=v_init  Measurements=None
      settings: SourceProductName=Simscape Electrical
  i : powerlib/Measurements/Current Measurement  PhasorSimulation=off  OutputType=Complex  PSBequivalent=0
      settings: SourceProductName=Simscape Electrical
  i_leak : powerlib/Measurements/Current Measurement  PhasorSimulation=off  OutputType=Complex  PSBequivalent=0
      settings: SourceProductName=Simscape Electrical
  v^2/R : Fcn  Expr=u^2/r_esr
  v_cap : powerlib/Measurements/Voltage Measurement  PhasorSimulation=off  OutputType=Complex  PSBequivalent=0
      settings: SourceProductName=Simscape Electrical
  v_r : powerlib/Measurements/Voltage Measurement  PhasorSimulation=off  OutputType=Complex  PSBequivalent=0
      settings: SourceProductName=Simscape Electrical
  VCC_in : PMIOPort  Side=Left
  VSS_in : PMIOPort  Port=2  Side=Left
  VCC_out : PMIOPort  Tag=PMCPort  Port=3  Side=Right
  VSS_out : PMIOPort  Tag=PMCPort  Port=4  Side=Right
  v_r_out : Outport
  v_cap_out : Outport  Port=2
  i_leak_out : Outport  Port=3
  p_chg_out : Outport  Port=4
  p_leak_out : Outport  Port=5
  i_out : Outport  Port=6
  c_out : Outport  Port=7
  r_out : Outport  Port=8
  r_leak_out : Outport  Port=9
  l_out : Outport  Port=10
  wires:
  i_leak/1 -> Mux2/1
  v_r/1 -> Mux1/1, v^2/R/1
  Mux6/1 -> c_out/1
  Mux7/1 -> r_out/1
  Mux8/1 -> r_leak_out/1
  Mux9/1 -> l_out/1
  Constant/1 -> Mux6/1
  Constant4/1 -> Mux7/1
  Constant5/1 -> Mux8/1
  ? -> Mux9/1
  c_in/1 -> Mux6/2
  l_in/1 -> Mux9/2
  r_leak_in/1 -> Mux8/2
  r_in/1 -> Mux7/2
  p_chg_in/1 -> Mux3/2
  Mux3/1 -> p_chg_out/1
  v_r_in/1 -> Mux1/2
  Mux1/1 -> v_r_out/1
  v^2/R/1 -> Mux3/1
  Mux2/1 -> i_leak_out/1
  i_leak_in/1 -> Mux2/2
  i/1 -> Mux5/1
  Mux5/1 -> i_out/1
  i_in/1 -> Mux5/2
  p_leak_in/1 -> Mux4/2
  Mux4/1 -> p_leak_out/1
  Mux/1 -> v_cap_out/1
  v_cap_in/1 -> Mux/2
  v_cap/1 -> Fcn1/1, Mux/1
  Fcn1/1 -> Mux4/1
  connections:
  Parallel RLC Branch1/RConn1 -- i_leak/LConn1
  VSS_out/RConn1 -- VSS_in/RConn1 -- i_leak/RConn1 -- Parallel RLC Branch11/RConn1 -- v_cap/LConn2
  Parallel RLC Branch1/LConn1 -- i/RConn1 -- Parallel RLC Branch11/LConn1 -- v_cap/LConn1
  VCC_out/RConn1 -- v_r/LConn1 -- Parallel RLC Branch10/LConn1 -- VCC_in/RConn1
  v_r/LConn2 -- i/LConn1 -- Parallel RLC Branch10/RConn1

== system cap_eq_circuit_pascal5_single_shot/Eq Circuit Network/Subsystem8 ==
  note: Export user input data
  Constant : Constant  Value=c
  Constant4 : Constant  Value=r_esr
  Constant5 : Constant  Value=r_leak
  Fcn1 : Fcn  Expr=u^2/r_leak
  Parallel RLC Branch1 : powerlib/Elements/Parallel RLC Branch  LConnTagsString=a  RConnTagsString=__new0  BranchType=R  Resistance=r_leak  Inductance=1e-3  SetiL0=off  InitialCurrent=0  Capacitance=1e-6  Setx0=off  InitialVoltage=0  Measurements=None
      settings: SourceProductName=Simscape Electrical
  Parallel RLC Branch10 : powerlib/Elements/Parallel RLC Branch  LConnTagsString=a  RConnTagsString=__new0  BranchType=R  Resistance=r_esr  Inductance=1e-3  SetiL0=off  InitialCurrent=0  Capacitance=1e-6  Setx0=off  InitialVoltage=0  Measurements=None
      settings: SourceProductName=Simscape Electrical
  Parallel RLC Branch11 : powerlib/Elements/Parallel RLC Branch  LConnTagsString=a  RConnTagsString=__new0  BranchType=C  Resistance=1  Inductance=1e-3  SetiL0=off  InitialCurrent=0  Capacitance=c  Setx0=on  InitialVoltage=v_init  Measurements=None
      settings: SourceProductName=Simscape Electrical
  i : powerlib/Measurements/Current Measurement  PhasorSimulation=off  OutputType=Complex  PSBequivalent=0
      settings: SourceProductName=Simscape Electrical
  i_leak : powerlib/Measurements/Current Measurement  PhasorSimulation=off  OutputType=Complex  PSBequivalent=0
      settings: SourceProductName=Simscape Electrical
  v^2/R : Fcn  Expr=u^2/r_esr
  v_cap : powerlib/Measurements/Voltage Measurement  PhasorSimulation=off  OutputType=Complex  PSBequivalent=0
      settings: SourceProductName=Simscape Electrical
  v_r : powerlib/Measurements/Voltage Measurement  PhasorSimulation=off  OutputType=Complex  PSBequivalent=0
      settings: SourceProductName=Simscape Electrical
  VCC_in : PMIOPort  Side=Left
  VSS_in : PMIOPort  Port=2  Side=Left
  VCC_out : PMIOPort  Tag=PMCPort  Port=3  Side=Right
  VSS_out : PMIOPort  Tag=PMCPort  Port=4  Side=Right
  v_r_out : Outport
  v_cap_out : Outport  Port=2
  i_leak_out : Outport  Port=3
  p_chg_out : Outport  Port=4
  p_leak_out : Outport  Port=5
  i_out : Outport  Port=6
  c_out : Outport  Port=7
  r_out : Outport  Port=8
  r_leak_out : Outport  Port=9
  l_out : Outport  Port=10
  wires:
  i_leak/1 -> i_leak_out/1
  v_r/1 -> v_r_out/1, v^2/R/1
  Constant/1 -> c_out/1
  Constant4/1 -> r_out/1
  Constant5/1 -> r_leak_out/1
  ? -> l_out/1
  i/1 -> i_out/1
  v_cap/1 -> v_cap_out/1, Fcn1/1
  Fcn1/1 -> p_leak_out/1
  v^2/R/1 -> p_chg_out/1
  connections:
  Parallel RLC Branch11/RConn1 -- v_cap/LConn2 -- i_leak/RConn1 -- VSS_out/RConn1 -- VSS_in/RConn1
  Parallel RLC Branch11/LConn1 -- Parallel RLC Branch1/LConn1 -- i/RConn1 -- v_cap/LConn1
  VCC_in/RConn1 -- VCC_out/RConn1 -- Parallel RLC Branch10/LConn1 -- v_r/LConn1
  Parallel RLC Branch10/RConn1 -- v_r/LConn2 -- i/LConn1
  Parallel RLC Branch1/RConn1 -- i_leak/LConn1

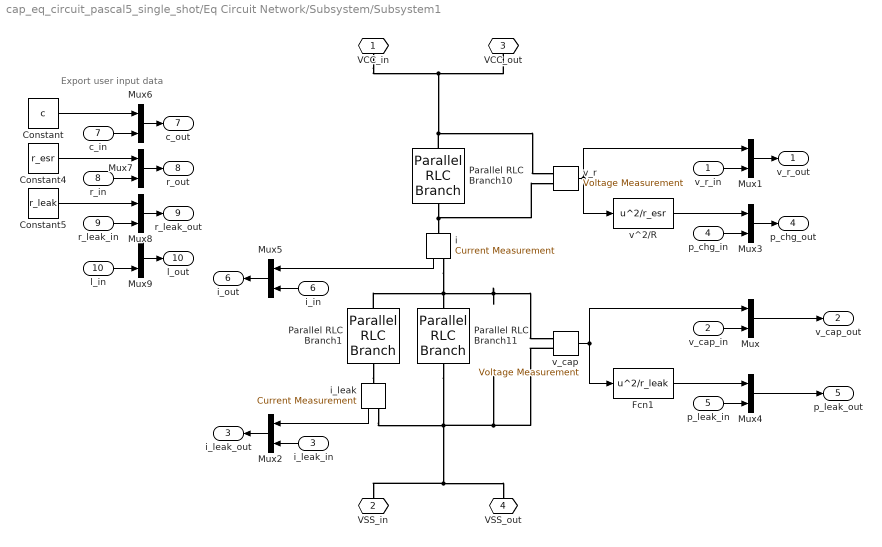
== system cap_eq_circuit_pascal5_single_shot/Eq Circuit Network/Subsystem/Subsystem1 ==
  note: Export user input data
  v_r_in : Inport
  v_cap_in : Inport  Port=2
  i_leak_in : Inport  Port=3
  p_chg_in : Inport  Port=4
  p_leak_in : Inport  Port=5
  i_in : Inport  Port=6
  c_in : Inport  Port=7
  r_in : Inport  Port=8
  r_leak_in : Inport  Port=9
  l_in : Inport  Port=10
  Constant : Constant  Value=c
  Constant4 : Constant  Value=r_esr
  Constant5 : Constant  Value=r_leak
  Fcn1 : Fcn  Expr=u^2/r_leak
  Mux{,1..9} (10 alike) : Mux  Inputs=2
  Parallel RLC Branch1 : powerlib/Elements/Parallel RLC Branch  LConnTagsString=a  RConnTagsString=__new0  BranchType=R  Resistance=r_leak  Inductance=1e-3  SetiL0=off  InitialCurrent=0  Capacitance=1e-6  Setx0=off  InitialVoltage=0  Measurements=None
      settings: SourceProductName=Simscape Electrical
  Parallel RLC Branch10 : powerlib/Elements/Parallel RLC Branch  LConnTagsString=a  RConnTagsString=__new0  BranchType=R  Resistance=r_esr  Inductance=1e-3  SetiL0=off  InitialCurrent=0  Capacitance=1e-6  Setx0=off  InitialVoltage=0  Measurements=None
      settings: SourceProductName=Simscape Electrical
  Parallel RLC Branch11 : powerlib/Elements/Parallel RLC Branch  LConnTagsString=a  RConnTagsString=__new0  BranchType=C  Resistance=1  Inductance=1e-3  SetiL0=off  InitialCurrent=0  Capacitance=c  Setx0=on  InitialVoltage=v_init  Measurements=None
      settings: SourceProductName=Simscape Electrical
  i : powerlib/Measurements/Current Measurement  PhasorSimulation=off  OutputType=Complex  PSBequivalent=0
      settings: SourceProductName=Simscape Electrical
  i_leak : powerlib/Measurements/Current Measurement  PhasorSimulation=off  OutputType=Complex  PSBequivalent=0
      settings: SourceProductName=Simscape Electrical
  v^2/R : Fcn  Expr=u^2/r_esr
  v_cap : powerlib/Measurements/Voltage Measurement  PhasorSimulation=off  OutputType=Complex  PSBequivalent=0
      settings: SourceProductName=Simscape Electrical
  v_r : powerlib/Measurements/Voltage Measurement  PhasorSimulation=off  OutputType=Complex  PSBequivalent=0
      settings: SourceProductName=Simscape Electrical
  VCC_in : PMIOPort  Side=Left
  VSS_in : PMIOPort  Port=2  Side=Left
  VCC_out : PMIOPort  Tag=PMCPort  Port=3  Side=Right
  VSS_out : PMIOPort  Tag=PMCPort  Port=4  Side=Right
  v_r_out : Outport
  v_cap_out : Outport  Port=2
  i_leak_out : Outport  Port=3
  p_chg_out : Outport  Port=4
  p_leak_out : Outport  Port=5
  i_out : Outport  Port=6
  c_out : Outport  Port=7
  r_out : Outport  Port=8
  r_leak_out : Outport  Port=9
  l_out : Outport  Port=10
  wires:
  Fcn1/1 -> Mux4/1
  v_cap/1 -> Mux/1, Fcn1/1
  v_cap_in/1 -> Mux/2
  Mux/1 -> v_cap_out/1
  Mux4/1 -> p_leak_out/1
  p_leak_in/1 -> Mux4/2
  i_in/1 -> Mux5/2
  Mux5/1 -> i_out/1
  i/1 -> Mux5/1
  i_leak_in/1 -> Mux2/2
  Mux2/1 -> i_leak_out/1
  v^2/R/1 -> Mux3/1
  Mux1/1 -> v_r_out/1
  v_r_in/1 -> Mux1/2
  Mux3/1 -> p_chg_out/1
  p_chg_in/1 -> Mux3/2
  r_in/1 -> Mux7/2
  r_leak_in/1 -> Mux8/2
  l_in/1 -> Mux9/2
  c_in/1 -> Mux6/2
  ? -> Mux9/1
  Constant5/1 -> Mux8/1
  Constant4/1 -> Mux7/1
  Constant/1 -> Mux6/1
  Mux9/1 -> l_out/1
  Mux8/1 -> r_leak_out/1
  Mux7/1 -> r_out/1
  Mux6/1 -> c_out/1
  v_r/1 -> v^2/R/1, Mux1/1
  i_leak/1 -> Mux2/1
  connections:
  Parallel RLC Branch10/RConn1 -- i/LConn1 -- v_r/LConn2
  VCC_in/RConn1 -- Parallel RLC Branch10/LConn1 -- v_r/LConn1 -- VCC_out/RConn1
  Parallel RLC Branch1/LConn1 -- Parallel RLC Branch11/LConn1 -- i/RConn1 -- v_cap/LConn1
  v_cap/LConn2 -- Parallel RLC Branch11/RConn1 -- i_leak/RConn1 -- VSS_in/RConn1 -- VSS_out/RConn1
  Parallel RLC Branch1/RConn1 -- i_leak/LConn1

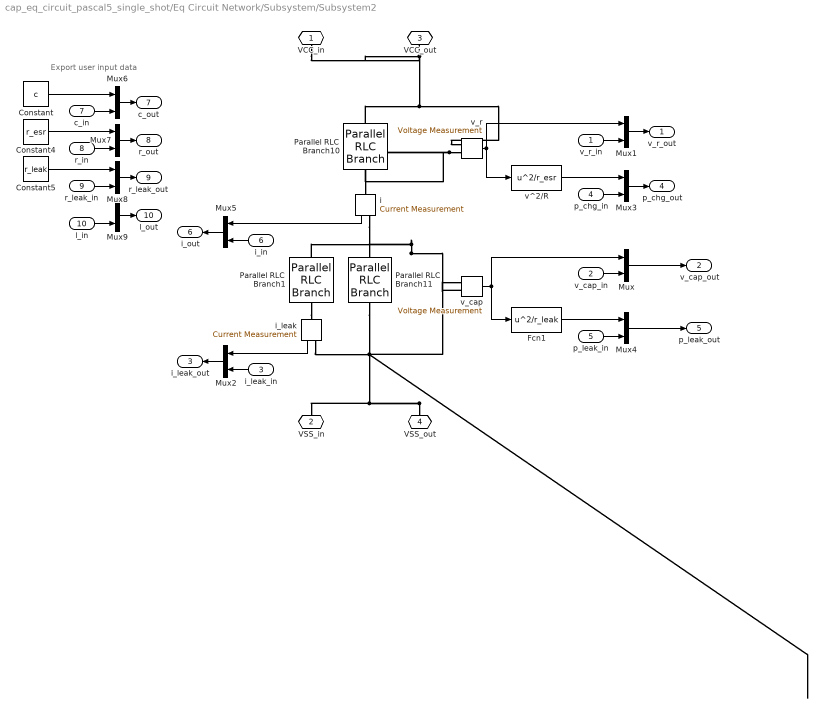
== system cap_eq_circuit_pascal5_single_shot/Eq Circuit Network/Subsystem/Subsystem2 ==
  note: Export user input data
  v_r_in : Inport
  v_cap_in : Inport  Port=2
  i_leak_in : Inport  Port=3
  p_chg_in : Inport  Port=4
  p_leak_in : Inport  Port=5
  i_in : Inport  Port=6
  c_in : Inport  Port=7
  r_in : Inport  Port=8
  r_leak_in : Inport  Port=9
  l_in : Inport  Port=10
  Constant : Constant  Value=c
  Constant4 : Constant  Value=r_esr
  Constant5 : Constant  Value=r_leak
  Fcn1 : Fcn  Expr=u^2/r_leak
  Mux{,1..9} (10 alike) : Mux  Inputs=2
  Parallel RLC Branch1 : powerlib/Elements/Parallel RLC Branch  LConnTagsString=a  RConnTagsString=__new0  BranchType=R  Resistance=r_leak  Inductance=1e-3  SetiL0=off  InitialCurrent=0  Capacitance=1e-6  Setx0=off  InitialVoltage=0  Measurements=None
      settings: SourceProductName=Simscape Electrical
  Parallel RLC Branch10 : powerlib/Elements/Parallel RLC Branch  LConnTagsString=a  RConnTagsString=__new0  BranchType=R  Resistance=r_esr  Inductance=1e-3  SetiL0=off  InitialCurrent=0  Capacitance=1e-6  Setx0=off  InitialVoltage=0  Measurements=None
      settings: SourceProductName=Simscape Electrical
  Parallel RLC Branch11 : powerlib/Elements/Parallel RLC Branch  LConnTagsString=a  RConnTagsString=__new0  BranchType=C  Resistance=1  Inductance=1e-3  SetiL0=off  InitialCurrent=0  Capacitance=c  Setx0=on  InitialVoltage=v_init  Measurements=None
      settings: SourceProductName=Simscape Electrical
  i : powerlib/Measurements/Current Measurement  PhasorSimulation=off  OutputType=Complex  PSBequivalent=0
      settings: SourceProductName=Simscape Electrical
  i_leak : powerlib/Measurements/Current Measurement  PhasorSimulation=off  OutputType=Complex  PSBequivalent=0
      settings: SourceProductName=Simscape Electrical
  v^2/R : Fcn  Expr=u^2/r_esr
  v_cap : powerlib/Measurements/Voltage Measurement  PhasorSimulation=off  OutputType=Complex  PSBequivalent=0
      settings: SourceProductName=Simscape Electrical
  v_r : powerlib/Measurements/Voltage Measurement  PhasorSimulation=off  OutputType=Complex  PSBequivalent=0
      settings: SourceProductName=Simscape Electrical
  VCC_in : PMIOPort  Side=Left
  VSS_in : PMIOPort  Port=2  Side=Left
  VCC_out : PMIOPort  Tag=PMCPort  Port=3  Side=Right
  VSS_out : PMIOPort  Tag=PMCPort  Port=4  Side=Right
  v_r_out : Outport
  v_cap_out : Outport  Port=2
  i_leak_out : Outport  Port=3
  p_chg_out : Outport  Port=4
  p_leak_out : Outport  Port=5
  i_out : Outport  Port=6
  c_out : Outport  Port=7
  r_out : Outport  Port=8
  r_leak_out : Outport  Port=9
  l_out : Outport  Port=10
  wires:
  i_leak/1 -> Mux2/1
  v_r/1 -> Mux1/1, v^2/R/1
  Mux6/1 -> c_out/1
  Mux7/1 -> r_out/1
  Mux8/1 -> r_leak_out/1
  Mux9/1 -> l_out/1
  Constant/1 -> Mux6/1
  Constant4/1 -> Mux7/1
  Constant5/1 -> Mux8/1
  ? -> Mux9/1
  c_in/1 -> Mux6/2
  l_in/1 -> Mux9/2
  r_leak_in/1 -> Mux8/2
  r_in/1 -> Mux7/2
  p_chg_in/1 -> Mux3/2
  Mux3/1 -> p_chg_out/1
  v_r_in/1 -> Mux1/2
  Mux1/1 -> v_r_out/1
  v^2/R/1 -> Mux3/1
  Mux2/1 -> i_leak_out/1
  i_leak_in/1 -> Mux2/2
  i/1 -> Mux5/1
  Mux5/1 -> i_out/1
  i_in/1 -> Mux5/2
  p_leak_in/1 -> Mux4/2
  Mux4/1 -> p_leak_out/1
  Mux/1 -> v_cap_out/1
  v_cap_in/1 -> Mux/2
  v_cap/1 -> Fcn1/1, Mux/1
  Fcn1/1 -> Mux4/1
  connections:
  Parallel RLC Branch1/RConn1 -- i_leak/LConn1
  VSS_out/RConn1 -- VSS_in/RConn1 -- i_leak/RConn1 -- Parallel RLC Branch11/RConn1 -- v_cap/LConn2
  v_cap/LConn1 -- i/RConn1 -- Parallel RLC Branch11/LConn1 -- Parallel RLC Branch1/LConn1
  VCC_out/RConn1 -- v_r/LConn1 -- Parallel RLC Branch10/LConn1 -- VCC_in/RConn1
  v_r/LConn2 -- i/LConn1 -- Parallel RLC Branch10/RConn1

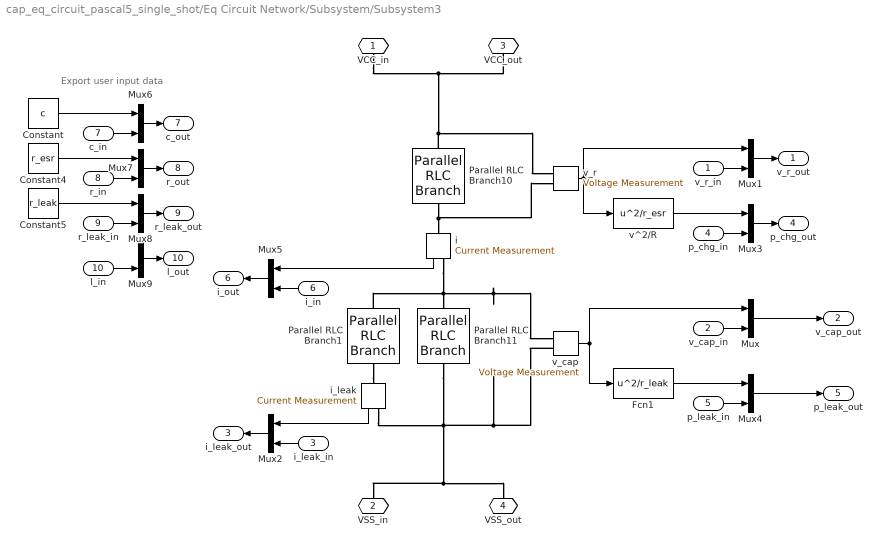
== system cap_eq_circuit_pascal5_single_shot/Eq Circuit Network/Subsystem/Subsystem3 ==
  note: Export user input data
  v_r_in : Inport
  v_cap_in : Inport  Port=2
  i_leak_in : Inport  Port=3
  p_chg_in : Inport  Port=4
  p_leak_in : Inport  Port=5
  i_in : Inport  Port=6
  c_in : Inport  Port=7
  r_in : Inport  Port=8
  r_leak_in : Inport  Port=9
  l_in : Inport  Port=10
  Constant : Constant  Value=c
  Constant4 : Constant  Value=r_esr
  Constant5 : Constant  Value=r_leak
  Fcn1 : Fcn  Expr=u^2/r_leak
  Mux{,1..9} (10 alike) : Mux  Inputs=2
  Parallel RLC Branch1 : powerlib/Elements/Parallel RLC Branch  LConnTagsString=a  RConnTagsString=__new0  BranchType=R  Resistance=r_leak  Inductance=1e-3  SetiL0=off  InitialCurrent=0  Capacitance=1e-6  Setx0=off  InitialVoltage=0  Measurements=None
      settings: SourceProductName=Simscape Electrical
  Parallel RLC Branch10 : powerlib/Elements/Parallel RLC Branch  LConnTagsString=a  RConnTagsString=__new0  BranchType=R  Resistance=r_esr  Inductance=1e-3  SetiL0=off  InitialCurrent=0  Capacitance=1e-6  Setx0=off  InitialVoltage=0  Measurements=None
      settings: SourceProductName=Simscape Electrical
  Parallel RLC Branch11 : powerlib/Elements/Parallel RLC Branch  LConnTagsString=a  RConnTagsString=__new0  BranchType=C  Resistance=1  Inductance=1e-3  SetiL0=off  InitialCurrent=0  Capacitance=c  Setx0=on  InitialVoltage=v_init  Measurements=None
      settings: SourceProductName=Simscape Electrical
  i : powerlib/Measurements/Current Measurement  PhasorSimulation=off  OutputType=Complex  PSBequivalent=0
      settings: SourceProductName=Simscape Electrical
  i_leak : powerlib/Measurements/Current Measurement  PhasorSimulation=off  OutputType=Complex  PSBequivalent=0
      settings: SourceProductName=Simscape Electrical
  v^2/R : Fcn  Expr=u^2/r_esr
  v_cap : powerlib/Measurements/Voltage Measurement  PhasorSimulation=off  OutputType=Complex  PSBequivalent=0
      settings: SourceProductName=Simscape Electrical
  v_r : powerlib/Measurements/Voltage Measurement  PhasorSimulation=off  OutputType=Complex  PSBequivalent=0
      settings: SourceProductName=Simscape Electrical
  VCC_in : PMIOPort  Side=Left
  VSS_in : PMIOPort  Port=2  Side=Left
  VCC_out : PMIOPort  Tag=PMCPort  Port=3  Side=Right
  VSS_out : PMIOPort  Tag=PMCPort  Port=4  Side=Right
  v_r_out : Outport
  v_cap_out : Outport  Port=2
  i_leak_out : Outport  Port=3
  p_chg_out : Outport  Port=4
  p_leak_out : Outport  Port=5
  i_out : Outport  Port=6
  c_out : Outport  Port=7
  r_out : Outport  Port=8
  r_leak_out : Outport  Port=9
  l_out : Outport  Port=10
  wires:
  Fcn1/1 -> Mux4/1
  v_cap/1 -> Mux/1, Fcn1/1
  v_cap_in/1 -> Mux/2
  Mux/1 -> v_cap_out/1
  Mux4/1 -> p_leak_out/1
  p_leak_in/1 -> Mux4/2
  i_in/1 -> Mux5/2
  Mux5/1 -> i_out/1
  i/1 -> Mux5/1
  i_leak_in/1 -> Mux2/2
  Mux2/1 -> i_leak_out/1
  v^2/R/1 -> Mux3/1
  Mux1/1 -> v_r_out/1
  v_r_in/1 -> Mux1/2
  Mux3/1 -> p_chg_out/1
  p_chg_in/1 -> Mux3/2
  r_in/1 -> Mux7/2
  r_leak_in/1 -> Mux8/2
  l_in/1 -> Mux9/2
  c_in/1 -> Mux6/2
  ? -> Mux9/1
  Constant5/1 -> Mux8/1
  Constant4/1 -> Mux7/1
  Constant/1 -> Mux6/1
  Mux9/1 -> l_out/1
  Mux8/1 -> r_leak_out/1
  Mux7/1 -> r_out/1
  Mux6/1 -> c_out/1
  v_r/1 -> v^2/R/1, Mux1/1
  i_leak/1 -> Mux2/1
  connections:
  Parallel RLC Branch10/RConn1 -- i/LConn1 -- v_r/LConn2
  VCC_in/RConn1 -- Parallel RLC Branch10/LConn1 -- v_r/LConn1 -- VCC_out/RConn1
  Parallel RLC Branch1/LConn1 -- Parallel RLC Branch11/LConn1 -- i/RConn1 -- v_cap/LConn1
  v_cap/LConn2 -- Parallel RLC Branch11/RConn1 -- i_leak/RConn1 -- VSS_in/RConn1 -- VSS_out/RConn1
  Parallel RLC Branch1/RConn1 -- i_leak/LConn1
